simulink model "simple_PID"  (R2022b)
settings: Solver=VariableStepAuto  StartTime=0.0  StopTime=15  RelTol=1e-3
settings Model: Creator=giuli  LastModifiedBy=giuli

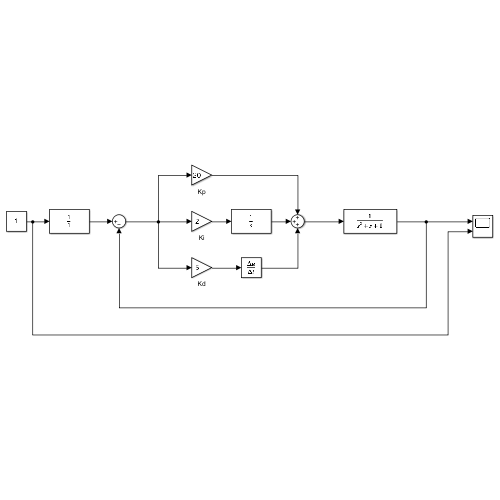
[thumbnail: Simulink's stored preview of the top-level diagram]
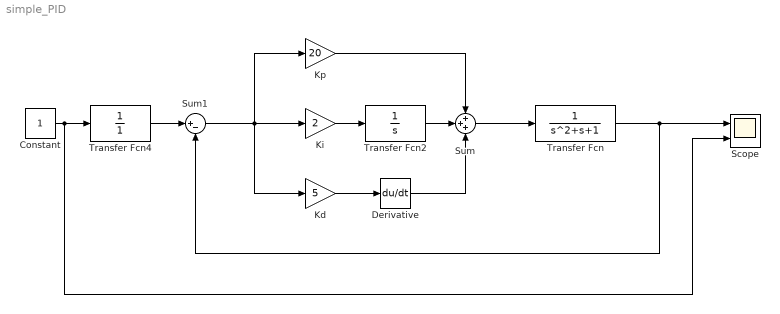
== system simple_PID ==
  Constant : Constant
  Derivative : Derivative
  Kd : Gain  Gain=5
  Ki : Gain  Gain=2
  Kp : Gain  Gain=20
  Scope : Scope  NumInputPorts=2
  Sum : Sum  Inputs=+++
  Sum1 : Sum  Inputs=|+-
  Transfer Fcn : TransferFcn  Denominator=[1 1 1]
  Transfer Fcn2 : TransferFcn  Denominator=[1 0]
  Transfer Fcn4 : TransferFcn  Numerator=1  Denominator=1
  wires:
  Transfer Fcn2/1 -> Sum/2
  Derivative/1 -> Sum/3
  Sum/1 -> Transfer Fcn/1
  Sum1/1 -> Kp/1, Kd/1, Ki/1
  Constant/1 -> Scope/2, Transfer Fcn4/1
  Transfer Fcn4/1 -> Sum1/1
  Transfer Fcn/1 -> Sum1/2, Scope/1
  Kp/1 -> Sum/1
  Ki/1 -> Transfer Fcn2/1
  Kd/1 -> Derivative/1
